simulink model "TrqCnv"  (R2018a)
settings: configuration reference "cs_ert" (kept outside this file)
settings Model: DataDictionary=TrqCnv.sldd  Creator=zhoutinglin  LastModifiedBy=zhoutinglin

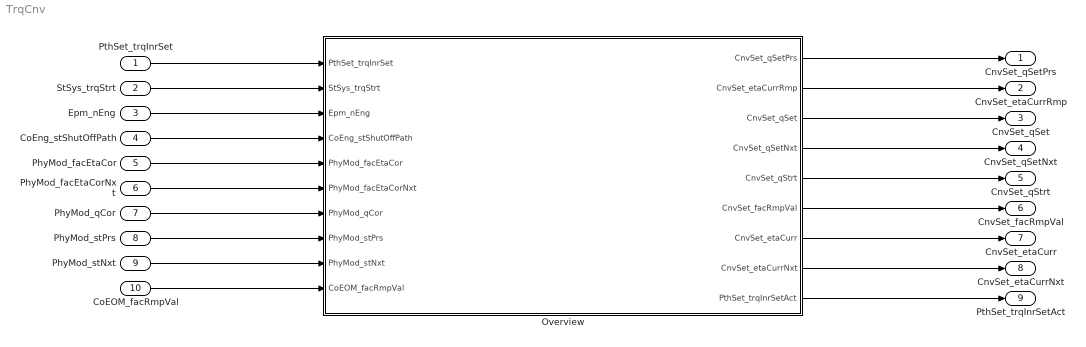
== system TrqCnv ==
  PthSet_trqInrSet : Inport
  StSys_trqStrt : Inport  Port=2
  Epm_nEng : Inport  Port=3
  CoEng_stShutOffPath : Inport  Port=4
  PhyMod_facEtaCor : Inport  Port=5
  PhyMod_facEtaCorNxt : Inport  Port=6
  PhyMod_qCor : Inport  Port=7
  PhyMod_stPrs : Inport  Port=8
  PhyMod_stNxt : Inport  Port=9
  CoEOM_facRmpVal : Inport  Port=10
  Overview : Subsystem
  CnvSet_qSetPrs : Outport
  CnvSet_etaCurrRmp : Outport  Port=2
  CnvSet_qSet : Outport  Port=3
  CnvSet_qSetNxt : Outport  Port=4
  CnvSet_qStrt : Outport  Port=5
  CnvSet_facRmpVal : Outport  Port=6
  CnvSet_etaCurr : Outport  Port=7
  CnvSet_etaCurrNxt : Outport  Port=8
  PthSet_trqInrSetAct : Outport  Port=9
  wires:
  PthSet_trqInrSet/1 -> Overview/1(PthSet_trqInrSet)
  StSys_trqStrt/1 -> Overview/2(StSys_trqStrt)
  Epm_nEng/1 -> Overview/3(Epm_nEng)
  CoEng_stShutOffPath/1 -> Overview/4(CoEng_stShutOffPath)
  PhyMod_facEtaCor/1 -> Overview/5(PhyMod_facEtaCor)
  PhyMod_facEtaCorNxt/1 -> Overview/6(PhyMod_facEtaCorNxt)
  PhyMod_qCor/1 -> Overview/7(PhyMod_qCor)
  PhyMod_stPrs/1 -> Overview/8(PhyMod_stPrs)
  PhyMod_stNxt/1 -> Overview/9(PhyMod_stNxt)
  CoEOM_facRmpVal/1 -> Overview/10(CoEOM_facRmpVal)
  Overview/1(CnvSet_qSetPrs) -> CnvSet_qSetPrs/1
  Overview/2(CnvSet_etaCurrRmp) -> CnvSet_etaCurrRmp/1
  Overview/3(CnvSet_qSet) -> CnvSet_qSet/1
  Overview/4(CnvSet_qSetNxt) -> CnvSet_qSetNxt/1
  Overview/5(CnvSet_qStrt) -> CnvSet_qStrt/1
  Overview/6(CnvSet_facRmpVal) -> CnvSet_facRmpVal/1
  Overview/7(CnvSet_etaCurr) -> CnvSet_etaCurr/1
  Overview/8(CnvSet_etaCurrNxt) -> CnvSet_etaCurrNxt/1
  Overview/9(PthSet_trqInrSetAct) -> PthSet_trqInrSetAct/1

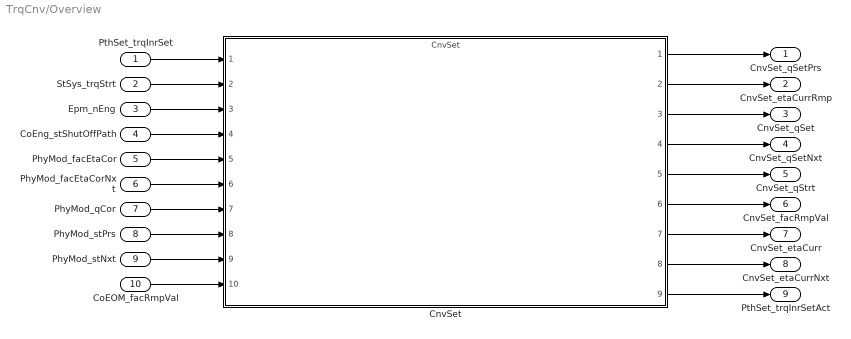
== system TrqCnv/Overview ==
  PthSet_trqInrSet : Inport
  StSys_trqStrt : Inport  Port=2
  Epm_nEng : Inport  Port=3
  CoEng_stShutOffPath : Inport  Port=4
  PhyMod_facEtaCor : Inport  Port=5
  PhyMod_facEtaCorNxt : Inport  Port=6
  PhyMod_qCor : Inport  Port=7
  PhyMod_stPrs : Inport  Port=8
  PhyMod_stNxt : Inport  Port=9
  CoEOM_facRmpVal : Inport  Port=10
  CnvSet : ModelReference  ModelNameDialog=CnvSet  SimulationMode=Normal  ModelReferenceVersion=1.2
  CnvSet_qSetPrs : Outport
  CnvSet_etaCurrRmp : Outport  Port=2
  CnvSet_qSet : Outport  Port=3
  CnvSet_qSetNxt : Outport  Port=4
  CnvSet_qStrt : Outport  Port=5
  CnvSet_facRmpVal : Outport  Port=6
  CnvSet_etaCurr : Outport  Port=7
  CnvSet_etaCurrNxt : Outport  Port=8
  PthSet_trqInrSetAct : Outport  Port=9
  wires:
  PthSet_trqInrSet/1 -> CnvSet/1
  StSys_trqStrt/1 -> CnvSet/2
  Epm_nEng/1 -> CnvSet/3
  CoEng_stShutOffPath/1 -> CnvSet/4
  PhyMod_facEtaCor/1 -> CnvSet/5
  PhyMod_facEtaCorNxt/1 -> CnvSet/6
  PhyMod_qCor/1 -> CnvSet/7
  PhyMod_stPrs/1 -> CnvSet/8
  PhyMod_stNxt/1 -> CnvSet/9
  CoEOM_facRmpVal/1 -> CnvSet/10
  CnvSet/1 -> CnvSet_qSetPrs/1
  CnvSet/2 -> CnvSet_etaCurrRmp/1
  CnvSet/3 -> CnvSet_qSet/1
  CnvSet/4 -> CnvSet_qSetNxt/1
  CnvSet/5 -> CnvSet_qStrt/1
  CnvSet/6 -> CnvSet_facRmpVal/1
  CnvSet/7 -> CnvSet_etaCurr/1
  CnvSet/8 -> CnvSet_etaCurrNxt/1
  CnvSet/9 -> PthSet_trqInrSetAct/1
